simulink model "automated_irrigation_control_system"  (R2023b)
settings: Solver=VariableStepAuto  StartTime=0.0  StopTime=10.0  RelTol=1e-3
libraries: simulink x2
settings Model: Creator=ascom  LastModifiedBy=ascom

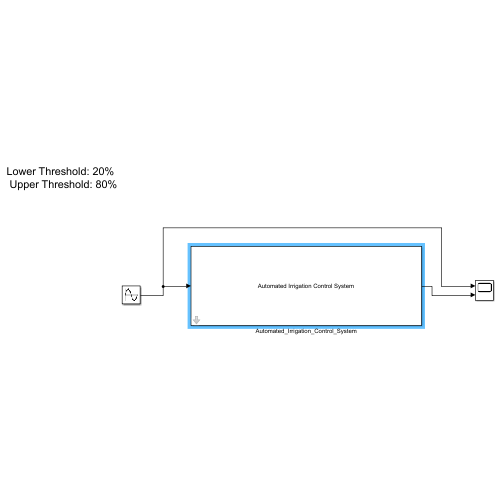
[thumbnail: Simulink's stored preview of the top-level diagram]
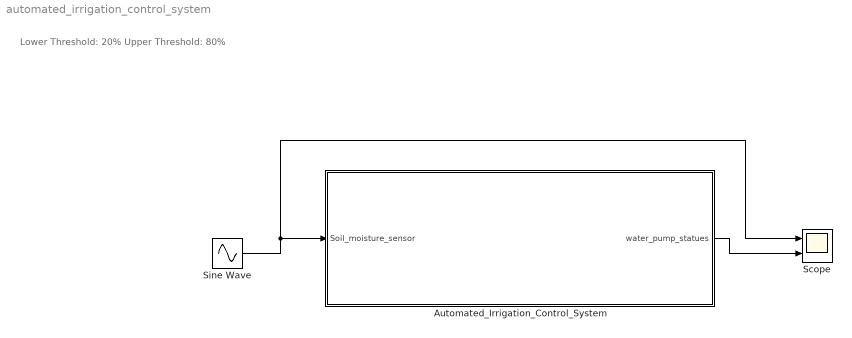
== system automated_irrigation_control_system ==
  note: Lower Threshold: 20%
      | Upper Threshold: 80%
  Automated_Irrigation_Control_System : Subsystem
      mask Display: disp('Automated Irrigation Control System');
  Scope : Scope  NumInputPorts=2
  Sine Wave : Sin  Amplitude=100  Frequency=2  SampleTime=0
  wires:
  Sine Wave/1 -> Scope/1, Automated_Irrigation_Control_System/1(Soil_moisture_sensor)
  Automated_Irrigation_Control_System/1(water_pump_statues) -> Scope/2

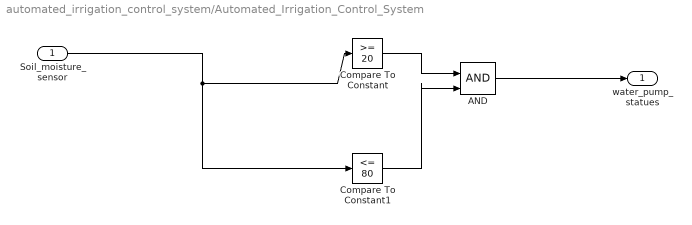
== system automated_irrigation_control_system/Automated_Irrigation_Control_System ==
  Soil_moisture_sensor : Inport
  AND : Logic  IconShape=distinctive  AllPortsSameDT=off  OutDataTypeStr=boolean
  Compare To Constant : simulink/Logic and Bit Operations/Compare To Constant  relop=>=  const=20  OutDataTypeStr=boolean
  Compare To Constant1 : simulink/Logic and Bit Operations/Compare To Constant  relop=<=  const=80  OutDataTypeStr=boolean
  water_pump_statues : Outport
  wires:
  Soil_moisture_sensor/1 -> Compare To Constant1/1, Compare To Constant/1
  Compare To Constant/1 -> AND/1
  Compare To Constant1/1 -> AND/2
  AND/1 -> water_pump_statues/1
